simulink model "PathTrackingVehicleController"  (R2026b)
settings: Solver=ode4  StopTime=10  FixedStep=0.01
model workspace (MAT data in the model file):
  PathTrackingAntiWindupGain = 0.5
  PathTrackingBrakePressurePerAcceleration = 10000
  PathTrackingControlSampleTime = 0.01
  PathTrackingCrossTrackGain = 2
  PathTrackingGearEfficiency = 0.95
  PathTrackingGearRatio = 10
  PathTrackingHeadingGain = 1.2
  PathTrackingMaximumAcceleration = 8
  PathTrackingMaximumDeceleration = 8
  PathTrackingMaximumSteeringAngle = 0.5
  PathTrackingMaximumSteeringRate = 4
  PathTrackingMinimumSteeringSpeed = 1
  PathTrackingMotorTorqueLimit = 40
  PathTrackingSpeedKi = 0.25
  PathTrackingSpeedKp = 0.8
  PathTrackingSteeringWheelRatio = 1
  PathTrackingTireEffectiveRadius = 0.23
  PathTrackingVehicleMass = 250
  PathTrackingWheelbase = 2
settings Model: DataDictionary=VehicleData.sldd  Creator=Xu Dingyi  LastModifiedBy=29358

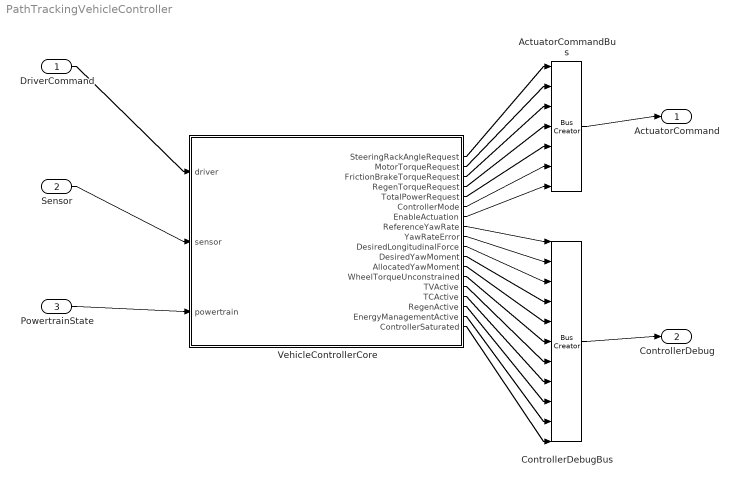
== system PathTrackingVehicleController ==
  DriverCommand : Inport  OutDataTypeStr=Bus: DriverCommandBus
  Sensor : Inport  Port=2  OutDataTypeStr=Bus: SensorBus
  PowertrainState : Inport  Port=3  OutDataTypeStr=Bus: PowertrainStateBus
  ActuatorCommandBus : BusCreator  Inputs=7  OutDataTypeStr=Bus: ActuatorCommandBus
  ControllerDebugBus : BusCreator  Inputs=11  OutDataTypeStr=Bus: ControllerDebugBus
  VehicleControllerCore : MATLAB Function  TreatAsAtomicUnit=on
  ActuatorCommand : Outport  OutDataTypeStr=Bus: ActuatorCommandBus
  ControllerDebug : Outport  Port=2  OutDataTypeStr=Bus: ControllerDebugBus
  wires:
  DriverCommand/1 -> VehicleControllerCore/1(driver)
  Sensor/1 -> VehicleControllerCore/2(sensor)
  PowertrainState/1 -> VehicleControllerCore/3(powertrain)
  VehicleControllerCore/1(SteeringRackAngleRequest) -> ActuatorCommandBus/1
  VehicleControllerCore/2(MotorTorqueRequest) -> ActuatorCommandBus/2
  VehicleControllerCore/3(FrictionBrakeTorqueRequest) -> ActuatorCommandBus/3
  VehicleControllerCore/4(RegenTorqueRequest) -> ActuatorCommandBus/4
  VehicleControllerCore/5(TotalPowerRequest) -> ActuatorCommandBus/5
  VehicleControllerCore/6(ControllerMode) -> ActuatorCommandBus/6
  VehicleControllerCore/7(EnableActuation) -> ActuatorCommandBus/7
  VehicleControllerCore/8(ReferenceYawRate) -> ControllerDebugBus/1
  VehicleControllerCore/9(YawRateError) -> ControllerDebugBus/2
  VehicleControllerCore/10(DesiredLongitudinalForce) -> ControllerDebugBus/3
  VehicleControllerCore/11(DesiredYawMoment) -> ControllerDebugBus/4
  VehicleControllerCore/12(AllocatedYawMoment) -> ControllerDebugBus/5
  VehicleControllerCore/13(WheelTorqueUnconstrained) -> ControllerDebugBus/6
  VehicleControllerCore/14(TVActive) -> ControllerDebugBus/7
  VehicleControllerCore/15(TCActive) -> ControllerDebugBus/8
  VehicleControllerCore/16(RegenActive) -> ControllerDebugBus/9
  VehicleControllerCore/17(EnergyManagementActive) -> ControllerDebugBus/10
  VehicleControllerCore/18(ControllerSaturated) -> ControllerDebugBus/11
  ActuatorCommandBus/1 -> ActuatorCommand/1
  ControllerDebugBus/1 -> ControllerDebug/1

== matlab function PathTrackingVehicleController/VehicleControllerCore ==
  data: driver input; SteeringRackAngleRequest output; sensor input; powertrain input; MotorTorqueRequest output; FrictionBrakeTorqueRequest output; RegenTorqueRequest output; TotalPowerRequest output; ControllerMode output; EnableActuation output; ReferenceYawRate output; YawRateError output; DesiredLongitudinalForce output; DesiredYawMoment output; AllocatedYawMoment output; WheelTorqueUnconstrained output; TVActive output; TCActive output; RegenActive output; EnergyManagementActive output; ControllerSaturated output; PathTrackingVehicleMass parameter double; PathTrackingTireEffectiveRadius parameter double; PathTrackingGearRatio parameter double; PathTrackingGearEfficiency parameter double; PathTrackingMotorTorqueLimit parameter double; PathTrackingMaximumAcceleration parameter double; PathTrackingMaximumDeceleration parameter double
function [SteeringRackAngleRequest, MotorTorqueRequest, ...
    FrictionBrakeTorqueRequest, RegenTorqueRequest, TotalPowerRequest, ...
    ControllerMode, EnableActuation, ReferenceYawRate, YawRateError, ...
    DesiredLongitudinalForce, DesiredYawMoment, AllocatedYawMoment, ...
    WheelTorqueUnconstrained, TVActive, TCActive, RegenActive, ...
    EnergyManagementActive, ControllerSaturated] = ...
    fcn(driver, sensor, powertrain, PathTrackingVehicleMass, PathTrackingTireEffectiveRadius, PathTrackingGearRatio, PathTrackingGearEfficiency, PathTrackingMotorTorqueLimit, PathTrackingMaximumAcceleration, PathTrackingMaximumDeceleration)
%FSAEPathTrackingVEHICLECONTROLLERCORE Baseline acceleration-to-four-motor allocator.

SteeringRackAngleRequest = driver.SteeringRackAngleRequest;
MotorTorqueRequest = zeros(4, 1);
FrictionBrakeTorqueRequest = zeros(4, 1);
RegenTorqueRequest = zeros(4, 1);
TotalPowerRequest = 0;
ControllerMode = uint8(0);
EnableActuation = false;
ReferenceYawRate = 0;
YawRateError = 0;
DesiredLongitudinalForce = 0;
DesiredYawMoment = 0;
AllocatedYawMoment = 0;
WheelTorqueUnconstrained = zeros(4, 1);
TVActive = false;
TCActive = false;
RegenActive = false;
EnergyManagementActive = false;
ControllerSaturated = false;

if driver.DriverMode == uint8(0) || ~sensor.PoseValid
    return
end
ControllerMode = uint8(2);
EnableActuation = driver.DriverMode == uint8(2);
TVActive = driver.EnableTV;
TCActive = driver.EnableTC;
RegenActive = driver.EnableRegen;
EnergyManagementActive = driver.EnableEnergyManagement;

DesiredLongitudinalForce = PathTrackingVehicleMass * ...
    min(PathTrackingMaximumAcceleration, max(-PathTrackingMaximumDeceleration, ...
    driver.LongitudinalAccelerationRequest));
WheelTorqueUnconstrained(:) = DesiredLongitudinalForce * ...
    PathTrackingTireEffectiveRadius / (4 * PathTrackingGearRatio * PathTrackingGearEfficiency);
MotorTorqueRequest(:) = min(PathTrackingMotorTorqueLimit, ...
    max(-PathTrackingMotorTorqueLimit, WheelTorqueUnconstrained));
ControllerSaturated = any(abs( ...
    MotorTorqueRequest - WheelTorqueUnconstrained) > 1.0e-9);

% Negative motor torque is the regenerative path.  Friction braking is added
% only for the residual force that the bounded motor torque cannot supply.
RegenTorqueRequest = max(0, -MotorTorqueRequest);
if ~RegenActive
    MotorTorqueRequest = max(0, MotorTorqueRequest);
    RegenTorqueRequest(:) = 0;
end
requestedBrakeForce = max(0, -DesiredLongitudinalForce);
availableRegenForce = sum(max(0, -MotorTorqueRequest)) * ...
    PathTrackingGearRatio * PathTrackingGearEfficiency / ...
    max(PathTrackingTireEffectiveRadius, 1.0e-6);
residualBrakeForce = max(0, requestedBrakeForce - availableRegenForce);
FrictionBrakeTorqueRequest(:) = residualBrakeForce * ...
    PathTrackingTireEffectiveRadius / 4;
ControllerSaturated = ControllerSaturated || residualBrakeForce > 1.0e-9;
TotalPowerRequest = sum(MotorTorqueRequest .* powertrain.MotorSpeed);
ReferenceYawRate = trackReferenceYawRate(driver, sensor);
YawRateError = ReferenceYawRate - sensor.YawRate;
end

function referenceYawRate = trackReferenceYawRate(driver, sensor)
% PathTracking DriverCommand does not carry curvature; the zero-yaw baseline is
% intentional until TV1 introduces a curvature/yaw reference bus.
referenceYawRate = 0;
if driver.DriverMode == uint8(2) && sensor.PoseValid
    referenceYawRate = 0;
end
end
